simulink model "Simulink_Sis_Rotacional"  (R2025a)
settings: Solver=VariableStepAuto  StartTime=0.0  StopTime=10.0  MaxStep=0.05  RelTol=1e-3
InitFcn:
  | m=10;
  | k=100;

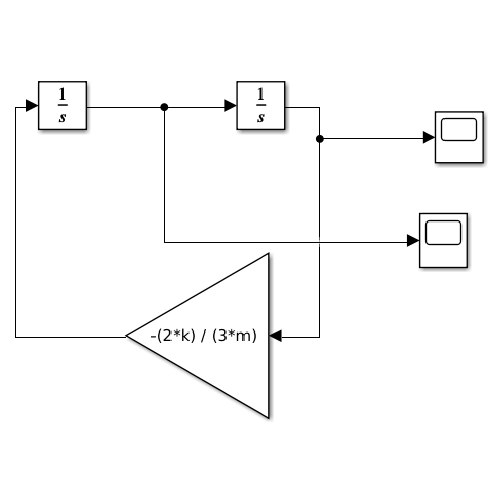
[thumbnail: Simulink's stored preview of the top-level diagram]
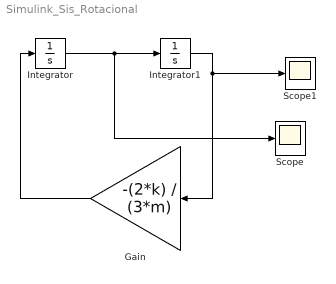
== system Simulink_Sis_Rotacional ==
  Gain : Gain  Gain=-(2*k) / (3*m)
  Integrator : Integrator  InitialCondition=2
  Integrator1 : Integrator
  Scope : Scope
      settings: ActiveDisplayYMinimum=-2.3996512908376784  ActiveDisplayYMaximum=2.476925130697444
  Scope1 : Scope
      settings: ActiveDisplayYMinimum=-1.0372780311773422  ActiveDisplayYMaximum=1.7769228141351592
  wires:
  Integrator/1 -> Scope/1, Integrator1/1
  Integrator1/1 -> Gain/1, Scope1/1
  Gain/1 -> Integrator/1
